simulink model "sf_slswitch"  (R2018b)
settings: Solver=ode45  StartTime=0.0  StopTime=options.T_train  MaxStep=.2  RelTol=1e-3  EnableMultiTasking=on
values from neighbouring files (symbols this model uses):
  options = trainingOptions('sgdm',      'MiniBatchSize',miniBatchSize,      'MaxEpochs',30,      'InitialLearnRate',1e-3,      'LearnRateSchedule','piecewise',      'LearnRateDropFactor',0.1,      'LearnRateDropPeriod',20,      'Shuffle','every-epoch',      'ValidationData',{XValidation,YValidation},      'ValidationFrequency',validationFrequency,      'Plots','training-progress',      'Verbose',false)    [training_lstm.m]
undefined symbols (not defined in the file or in its folder): DiscIntNeverNeededParam
libraries: simulink x3
settings Model: Creator=The MathWorks, Inc.  LastModifiedBy=kekatos
settings DataIOCC: LimitDataPoints=on  SaveFormat=Array
settings OptimizationCC: ExpressionDepthLimit=2147483647  LifeSpan=inf
settings DebuggingCC: UnderspecifiedInitializationDetection=Classic  MergeDetectMultiDrivingBlocksExec=none  SolverPrmCheckMsg=warning  FcnCallInpInsideContextMsg=warning  StateNameClashWarn=warning  LibraryContextMissingDiagnostic=none  SFUnexpectedBacktrackingDiag=warning  SFNoUnconditionalDefaultTransitionDiag=warning  SFExecutionAtInitializationDiag=none
settings HardwareCC: ProdBitPerPointer=32  ProdBitPerSizeT=32  ProdBitPerPtrDiffT=32  ProdLargestAtomicFloat=None  ProdIntDivRoundTo=Undefined  ProdEndianess=Unspecified  ProdWordSize=32  ProdHWDeviceType=32-bit Generic
settings ModelReferenceCC: PropagateSignalLabelsOutOfModel=off
settings SFSimCC: SimUseLocalCustomCode=off  SimParseCustomCode=off
settings RTWCC: RTWUseLocalCustomCode=off
settings CodeAppCC: StateflowObjectComments=on
settings GRTTargetCC: TargetLangStandard=C89/C90 (ANSI)  GeneratePreprocessorConditionals=Disable all  CombineOutputUpdateFcns=off  GRTInterface=on
settings ConfigComp: CovMetricSettings=dw  CovHtmlReporting=on  CovSaveCumulativeToWorkspaceVar=on  CovSaveSingleToWorkspaceVar=on  CovExternalEMLEnable=off  CovSFcnEnable=off

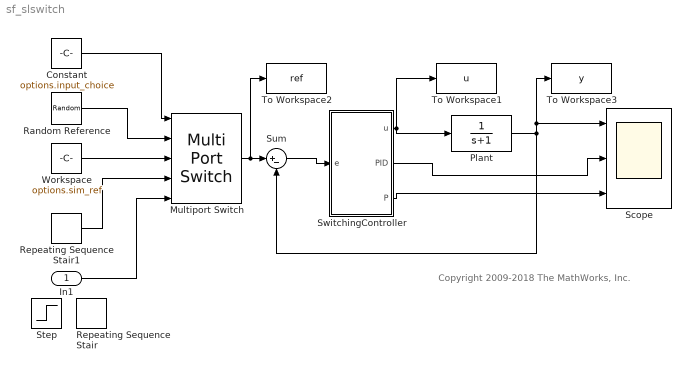
== system sf_slswitch ==
  note: Copyright 2009-2018 The MathWorks, Inc.
  In1 : Inport
  Constant : Constant  Value=options.input_choice
  Multiport Switch : MultiPortSwitch  Inputs=4
  Plant : TransferFcn  Denominator=[1 1]
  Random Reference : UniformRandomNumber  Minimum=options.ref_min  Maximum=options.ref_max  Seed=randi(2^32,[1 ])  SampleTime=options.ref_Ts
  Repeating Sequence Stair : simulink/Sources/Repeating Sequence Stair  OutValues=[1;2]  tsamp=10  OutMin=[]  OutMax=[]  OutDataTypeStr=double  OutputDataTypeScalingMode=double  OutDataType=fixdt(0,8)  ConRadixGroup=Best Precision: Vector-wise  OutScaling=2^-12
  Repeating Sequence Stair1 : simulink/Sources/Repeating Sequence Stair  OutValues=options.sim_cov  tsamp=options.ref_Ts  OutMin=[]  OutMax=[]  OutDataTypeStr=double  OutputDataTypeScalingMode=double  OutDataType=fixdt(0,8)  ConRadixGroup=Best Precision: Vector-wise  OutScaling=2^-12
  Scope : Scope  NumInputPorts=3
  Step : Step  Time=0  After=2  SampleTime=0
  Sum : Sum  Inputs=|+-
  SwitchingController : Stateflow chart  TreatAsAtomicUnit=on
  To Workspace1 : ToWorkspace  VariableName=u  SaveFormat=Structure With Time  SampleTime=options.dt
  To Workspace2 : ToWorkspace  VariableName=ref  SaveFormat=Structure With Time  SampleTime=options.dt
  To Workspace3 : ToWorkspace  VariableName=y  SaveFormat=Structure With Time  SampleTime=options.dt
  Workspace : Constant  Value=options.sim_ref
  wires:
  Sum/1 -> SwitchingController/1(e)
  Plant/1 -> Sum/2, To Workspace3/1, Scope/1
  SwitchingController/2(" PID") -> Scope/2
  SwitchingController/3(P) -> Scope/3
  Workspace/1 -> Multiport Switch/3
  Random Reference/1 -> Multiport Switch/2
  Repeating Sequence Stair1/1 -> Multiport Switch/4
  Constant/1 -> Multiport Switch/1
  In1/1 -> Multiport Switch/5
  Multiport Switch/1 -> To Workspace2/1, Sum/1
  SwitchingController/1(u) -> To Workspace1/1, Plant/1

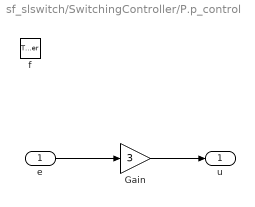
== system sf_slswitch/SwitchingController/P.p_control ==
  e : Inport
  f : TriggerPort  TriggerType=function-call  VariantControl=(inherit)
      settings: CopyFcn=Stateflow.SLINSF.SimulinkMan.removeBlockPreDeleteFcn  PreDeleteFcn=Stateflow.SLINSF.SimulinkMan.unsafePredeleteFcn
  Gain : Gain  Gain=3
  u : Outport
  wires:
  e/1 -> Gain/1
  Gain/1 -> u/1

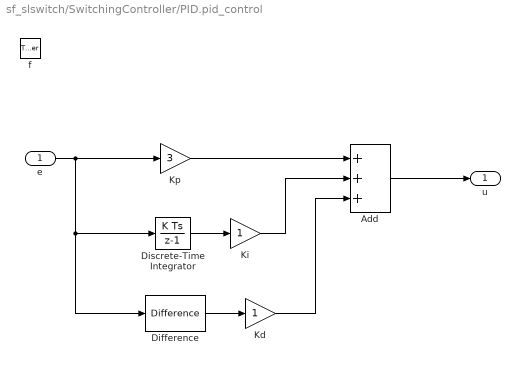
== system sf_slswitch/SwitchingController/PID.pid_control ==
  e : Inport
  f : TriggerPort  TriggerType=function-call  VariantControl=(inherit)
      settings: CopyFcn=Stateflow.SLINSF.SimulinkMan.removeBlockPreDeleteFcn  PreDeleteFcn=Stateflow.SLINSF.SimulinkMan.unsafePredeleteFcn
  Add : Sum  Inputs=+++
  Difference : simulink/Discrete/Difference  ICPrevInput=0.0  OutMin=[]  OutMax=[]  OutDataType=fixdt(1, 16)  OutScaling=2^-10  DoSatur=off
  Discrete-Time Integrator : DiscreteIntegrator  SampleTime=-1  ICPrevOutput=DiscIntNeverNeededParam  ICPrevScaledInput=DiscIntNeverNeededParam
  Kd : Gain
  Ki : Gain
  Kp : Gain  Gain=3
  u : Outport
  wires:
  e/1 -> Kp/1, Discrete-Time Integrator/1, Difference/1
  Kp/1 -> Add/1
  Add/1 -> u/1
  Discrete-Time Integrator/1 -> Ki/1
  Difference/1 -> Kd/1
  Ki/1 -> Add/2
  Kd/1 -> Add/3

== stateflow chart sf_slswitch/SwitchingController ==
  state STEADY
    entry: u = 0;
  state P
    du:
    u = p_control(e);
    state u = p_control(e) [function]
  state PID
    du:
    u = pid_control(e);
    state u = pid_control(e) [function]
  (default) -> STEADY
  STEADY -> P : [e > 0.01]
  P -> PID : [e < PID_TRESH]
  data: e function_input; u function_output; e function_input; u function_output; e input; u output double; PID output boolean; PID_TRESH parameter; P output boolean
